simulink model "p2_simulink"  (R2020a)
settings: Solver=VariableStepAuto  StartTime=0.0  StopTime=tsim  RelTol=1e-3
values from neighbouring files (symbols this model uses):
  fs = Spb*rb    (= 10000)    [p1_matlab.m]    (also in p2_matlab.m = 100000; p3_matlab.m = 100000; parte1.m = 100000; parte2.m = 100000)
  rb = 1000    [p1_matlab.m]    (also in p2_matlab.m; p3_matlab.m; parte1.m; parte2.m)
  Spb = 10    [p1_matlab.m]    (also in p2_matlab.m = 100; p3_matlab.m = 100; parte1.m = 100; parte2.m = 100)
libraries: commchan3 x1, commrandsrc3 x1, dspsigops x1, commutil2 x1
settings Model: Creator=pedro  LastModifiedBy=pedro

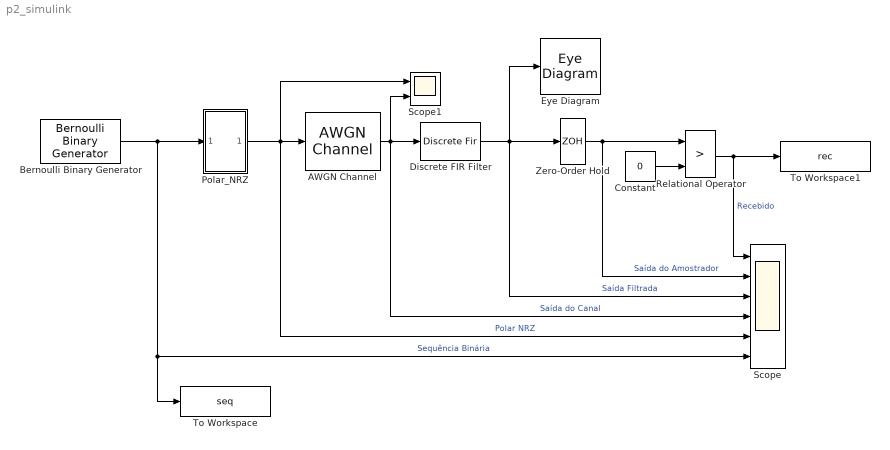
== system p2_simulink ==
  AWGN Channel : commchan3/AWGN Channel  InputProcessing=Columns as channels (frame based)  seed=0  noiseMode=Variance from mask  EbNodB=10  EsNodB=10  SNRdB=10  bitsPerSym=1  Ps=1  Tsym=1  variance=sigmaquadrado
  Bernoulli Binary Generator : commrandsrc3/Bernoulli Binary Generator  ProbabilityOfZero=0.5  SeedSource=Parameter  Seed=0  SampleTime=1/rb  SamplesPerFrame=1  OutputDataType=double  SimulateUsing=Interpreted execution
  Constant : Constant  Value=0
  Discrete FIR Filter : DiscreteFir  Coefficients=ones(1, 100)./100  SampleTime=1/fs
  Eye Diagram : EyeDiagram
  Polar_NRZ : Subsystem  mask(Polar_nrz){Rb=rb, Spb=Spb}
      mask prompts: Rb "Binary Data Rate"; Spb "Samples per bit"
  Relational Operator : RelationalOperator  Operator=>  OutDataTypeStr=boolean  RndMeth=Simplest
  Scope : Scope  NumInputPorts=6
  Scope1 : Scope  NumInputPorts=2
  To Workspace : ToWorkspace  VariableName=seq  SaveFormat=Timeseries  SampleTime=-1
  To Workspace1 : ToWorkspace  VariableName=rec  SaveFormat=Timeseries  SampleTime=-1
  Zero-Order Hold : ZeroOrderHold  SampleTime=1/rb
  wires:
  Constant/1 -> Relational Operator/2
  Polar_NRZ/1(Out1) -> AWGN Channel/1, Scope1/1, Scope/5  "Polar NRZ"
  Bernoulli Binary Generator/1 -> Scope/6, To Workspace/1, Polar_NRZ/1(In1)  "Sequência Binária"
  Relational Operator/1 -> To Workspace1/1, Scope/1  "Recebido"
  Zero-Order Hold/1 -> Scope/2, Relational Operator/1  "Saída do Amostrador"
  AWGN Channel/1 -> Scope1/2, Scope/4, Discrete FIR Filter/1  "Saída do Canal"
  Discrete FIR Filter/1 -> Eye Diagram/1, Scope/3, Zero-Order Hold/1  "Saída Filtrada"

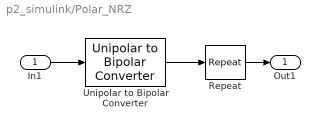
== system p2_simulink/Polar_NRZ ==
  In1 : Inport
  Repeat : dspsigops/Repeat  N=Spb  InputProcessing=Columns as channels (frame based)  RateOptions=Allow multirate processing  ic=0  mode=Unused parameter value
  Unipolar to Bipolar Converter : commutil2/Unipolar to Bipolar Converter  M=2  polarity=Positive  dataType=Same as input
  Out1 : Outport
  wires:
  Unipolar to Bipolar Converter/1 -> Repeat/1
  In1/1 -> Unipolar to Bipolar Converter/1
  Repeat/1 -> Out1/1
